simulink model "Lorenz_Simu"  (R2017b)
settings: Solver=VariableStepAuto  StartTime=0.0  StopTime=500  RelTol=1e-3
values from neighbouring files (symbols this model uses):
  b = 8/3    (= 2.66666666667)    [Lorenz.m]    (also in chua_integracion_numerica.m = 14)
  r = 28    [Lorenz.m]
  sig = 10    [Lorenz.m]
libraries: simulink x1
settings Model: Creator=franj  LastModifiedBy=gabri

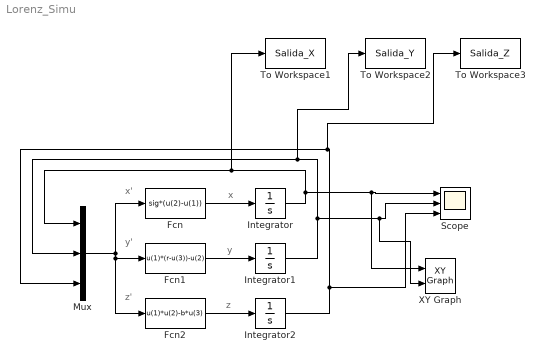
== system Lorenz_Simu ==
  note: x'
  note: y'
  note: z'
  note: x
  note: y
  note: z
  Fcn : Fcn  Expr=sig*(u(2)-u(1))
  Fcn1 : Fcn  Expr=u(1)*(r-u(3))-u(2)
  Fcn2 : Fcn  Expr=u(1)*u(2)-b*u(3)
  Integrator : Integrator  InitialCondition=1
  Integrator1 : Integrator  InitialCondition=1
  Integrator2 : Integrator  InitialCondition=1
  Mux : Mux  Inputs=3
  Scope : Scope  NumInputPorts=3
  To Workspace1 : ToWorkspace  VariableName=Salida_X  SampleTime=0.001
  To Workspace2 : ToWorkspace  VariableName=Salida_Y  SampleTime=0.001
  To Workspace3 : ToWorkspace  VariableName=Salida_Z  SampleTime=0.001
  XY Graph : simulink/Sinks/XY Graph  xmin=-20  xmax=20  ymin=-50  ymax=50  st=-1
  wires:
  Mux/1 -> Fcn1/1, Fcn2/1, Fcn/1
  Fcn2/1 -> Integrator2/1
  Fcn1/1 -> Integrator1/1
  Fcn/1 -> Integrator/1
  Integrator1/1 -> XY Graph/2, Scope/2, To Workspace2/1, Mux/2
  Integrator2/1 -> Scope/3, To Workspace3/1, Mux/3
  Integrator/1 -> XY Graph/1, Scope/1, To Workspace1/1, Mux/1
